simulink model "ModeSwitch_FLY"  (R2017b)
settings: Solver=FixedStepDiscrete  StartTime=0.0  StopTime=10.0  RelTol=1e-3
values from neighbouring files (symbols this model uses):
  DEG2RAD = 0.0174533    [Init_control.m]
  Kd_PITCH_AngleRate = 0.001    [Init_control.m]
  Kd_ROLL_AngleRate = 0.001    [Init_control.m]
  Kd_YAW_AngleRate = 0.00    (= 0)    [Init_control.m]
  Ki_PITCH_AngleRate = 0.02    [Init_control.m]
  Ki_ROLL_AngleRate = 0.02    [Init_control.m]
  Ki_YAW_AngleRate = 0.001    [Init_control.m]
  Kp_PITCH_ANGLE = 6.5    [Init_control.m]
  Kp_PITCH_AngleRate = 0.1    [Init_control.m]
  Kp_ROLL_ANGLE = 6.5    [Init_control.m]
  Kp_ROLL_AngleRate = 0.1    [Init_control.m]
  Kp_YAW_AngleRate = 0.3    [Init_control.m]
  Kpxp = 1.0    (= 1)    [Init_control.m]
  Kpyp = 1.0    (= 1)    [Init_control.m]
  Kpzp = 4.0    (= 4)    [Init_control.m]
  Kvxd = 0.01    [Init_control.m]
  Kvxi = 0.4    [Init_control.m]
  Kvxp = 2.5    [Init_control.m]
  Kvyd = 0.01    [Init_control.m]
  Kvyi = 0.4    [Init_control.m]
  Kvyp = 2.5    [Init_control.m]
  Kvzd = 0.005    [Init_control.m]
  Kvzi = 0.01    [Init_control.m]
  Kvzp = 0.45    [Init_control.m]
  MAX_CONTROL_ANGLE_PITCH = 35    [Init_control.m]
  MAX_CONTROL_ANGLE_RATE_PITCH = 220    [Init_control.m]
  MAX_CONTROL_ANGLE_RATE_ROLL = 220    [Init_control.m]
  MAX_CONTROL_ANGLE_RATE_Y = 200    [Init_control.m]
  MAX_CONTROL_ANGLE_ROLL = 35    [Init_control.m]
  MAX_CONTROL_VELOCITY_XY = 5    [Init_control.m]
  MAX_CONTROL_VELOCITY_Z = 3    [Init_control.m]
  Saturation_I_ah = 3.43    [Init_control.m]
  Saturation_I_az = 5    [Init_control.m]
  Saturation_I_RP_Max = 0.3    [Init_control.m]
  Saturation_I_RP_Min = -0.3    [Init_control.m]
  Saturation_I_Y_Max = 0.2    [Init_control.m]
  Saturation_I_Y_Min = -0.2    [Init_control.m]
  THR_HOVER = 0.609    [Init_control.m]
undefined symbols (not defined in the file or in its folder): DiscIntNeverNeededParam, RGBLED_COLOR_ENUM, RGBLED_MODE_ENUM
libraries: simulink x7, pixhawk_slib_sensors_actuators x5, pixhawk_slib_uORB_RW x1
settings Model: Creator=wsh  LastModifiedBy=Mr Wang
settings OptimizationCC: DefaultParameterBehavior=Inlined  MaxStackSize=64
settings DebuggingCC: ParameterTunabilityLossMsg=error
settings HardwareCC: ProdBitPerPointer=32  ProdBitPerSizeT=32  ProdBitPerPtrDiffT=32  ProdLargestAtomicInteger=Long  ProdLargestAtomicFloat=Double  ProdWordSize=32  ProdHWDeviceType=ARM Compatible->ARM Cortex
settings SFSimCC: MATLABDynamicMemAlloc=off
settings RTWCC: SystemTargetFile=ert.tlc  HardwareBoard=Pixhawk PX4  TemplateMakefile=ert_default_tmf  GenerateReport=on  Toolchain=Pixhawk Toolchain  IncludeHyperlinkInReport=on  LaunchReport=on  GenerateTraceInfo=on  GenerateTraceReport=on  GenerateTraceReportSl=on  GenerateTraceReportSf=on  GenerateTraceReportEml=on
settings CodeAppCC: ForceParamTrailComments=on  IgnoreCustomStorageClasses=off  OperatorAnnotations=on  SimulinkDataObjDesc=on  SFDataObjDesc=on  MATLABFcnDesc=on  InsertBlockDesc=on  StateflowObjectComments=on  MATLABSourceComments=on
settings ERTTargetCC: MultiwordLength=2048  ERTCustomFileTemplate=PX4_codertarget_file_process.tlc

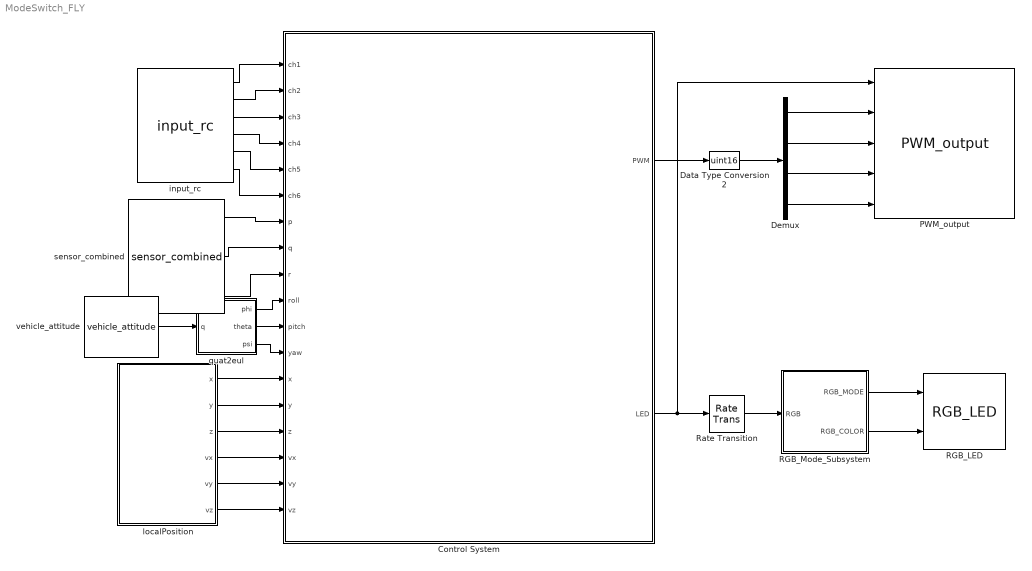
== system ModeSwitch_FLY ==
  Control System : Subsystem
      mask Display: image('icon\pixhawk.png');
  Data Type Conversion2 : DataTypeConversion  OutDataTypeStr=uint16
  Demux : Demux
  PWM_output : pixhawk_slib_sensors_actuators/PWM_output  Description=|  pub_outputs=on  pwm_rate=400Hz  show_pwm1=on  show_pwm5=off  show_pwm2=on  show_pwm6=off  show_pwm3=on  show_pwm7=off  show_pwm4=on  show_pwm8=off
      | This block allows the user to send the appropriate PWM signals out to the PX4 outputs.  
      | These are usually connected to the ESCs which control the motor speeds. 
      | In order for the flight control to arm (enable) the output from the software side, the ARM Output input must be held high (boolean TRUE).  
      | Only then will the PWM values be sent out the PX4 hardware ports.  
      | This is usually a function of the RC Tx in combination with other flight modes programmed in the Simulink model by the user.  
      | The block has 8 available ports (data type uint16) which can be selectively chosen.  
      | These correspond to the 8 PWM output ports on the px4fmu hardware.
      settings: SourceProductName=Pixhawk Target Blocks
  RGB_LED : pixhawk_slib_sensors_actuators/RGB_LED
      settings: SourceProductName=Pixhawk Target Blocks
  RGB_Mode_Subsystem : Subsystem
  Rate Transition : RateTransition  OutPortSampleTime=1
  input_rc : pixhawk_slib_sensors_actuators/input_rc  Description=|  sampletime=0.004  channel1=on  channel2=on  channel3=on  channel4=on  channel5=on  channel6=on  channel7=off  channel8=off  channel9=off  channel10=off  channel11=off  channel12=off  channel13=off  channel14=off  channel15=off  channel16=off  channel17=off  channel18=off  ch_count=off  rssi=off  rc_failsafe=off  rc_lost=off  rc_inputsource=off
      | RC Input Block
      | 
      | This block provides user input control to the model.
      | It uses the input_rc uORB topic.
      | 
      | The user has the ability to choose which channels are available as outputs from this block and also some optional outputs. These include 
      | Channels 1 through 18
      | double data type indicating the PWM value from the controller 
      | measured pulse widths for each of the supported channels 
      | Channel Count 
      | uint32 data type of the number of channels which are detector by the PX4 
      | RC Failsafe 
      | boolean data types indicating that the RC Tx is sending the FailSafe signal (if equipped and properly setup) 
      | explicit failsafe flag: true on TX failure or TX out of range , false otherwise. 
      | Only the true state is reliable, as there are some (PPM) receivers on the market going into failsafe without telling us explicitly. 
      | RC Input Source 
      | Enumeration data type indicating which source the RC input is from. 
      | Valid values are found in the ENUM file: RC_INPUT_SOURCE_ENUM.m 
      |           Enumeration members for class 'RC_INPUT_SOURCE_ENUM':
      |           RCINPUT_SOURCE_UNKNOWN         (0)
      |           RCINPUT_SOURCE_PX4FMU_PPM      (1)
      |           RCINPUT_SOURCE_PX4IO_PPM       (2)
      |           RCINPUT_SOURCE_PX4IO_SPEKTRUM  (3)
      |           RCINPUT_SOURCE_PX4IO_SBUS      (4)
      |           RCINPUT_SOURCE_PX4IO_ST24      (5)
      |           RCINPUT_SOURCE_MAVLINK         (6)
      |           RCINPUT_SOURCE_QURT            (7)
      |           RCINPUT_SOURCE_PX4FMU_SPEKTRUM (8)
      |           RCINPUT_SOURCE_PX4FMU_SBUS     (9)
      |           RCINPUT_SOURCE_PX4FMU_ST24     (10)
      |           RCINPUT_SOURCE_PX4FMU_SUMD     (11)
      |           RCINPUT_SOURCE_PX4FMU_DSM      (12)
      |           RCINPUT_SOURCE_PX4IO_SUMD      (13)
      | 
      | RSSI - Receive signal strength index 
      | receive signal strength indicator (RSSI): < 0: Undefined, 0: no signal, 255: full reception 
      | RC Lost Connection 
      | boolean data type indicating RC receiver connection status 
      | True, if no frame has arrived in the expected time, false otherwise. 
      | True usally means that the receiver has been disconnected, but can also indicate a radio link loss on "stupid" systems. 
      | Will remain false, if a RX with failsafe option continues to transmit frames after a link loss. 
      |   
      | Sample Model: px4demo_input_rc.slx
      settings: SourceProductName=Pixhawk Target Blocks
  "localPosition " : Subsystem
  quat2eul : MATLAB Function  TreatAsAtomicUnit=on
  sensor_combined : pixhawk_slib_sensors_actuators/sensor_combined  Description=|  sampletime=0.004  show_mag=off  show_acc=off  show_gyro=on  show_baro=off  show_ts=off
      | Sensor Combined Block
      | 
      | This block enables access to the various sensors available on the px4fmu-v2 hardware.  
      | The user can use these signals in the Simulink control model.  
      | The sample time needs to be provided in the mask dialog.  
      | Optional output ports can also be selected.  
      | Refer to the sample model: px4demo_attitude_control.slx
      | 
      | Signal definitions: 
      | Magnetometer (x,y,z) - single values – Magnetic field in NED body frame, in Gauss 
      | Accelerometer (x,y,z) - single values – Acceleration in NED body frame, in m/s^2 
      | Gyroscope (p,q,r) - single values – Angular velocity in radians per second 
      | Barometer (Altitude) - single value – Barometric pressure, already temperature compensated (millibars) 
      | RunTime (timestamp) - double value – Timestamp in microseconds since boot, from gyro 
      |   
      | The sensor_combined block needs to have the px4io service running on the PX4 hardware in order to get valid signal values.
      settings: SourceProductName=Pixhawk Target Blocks
  vehicle_attitude : pixhawk_slib_sensors_actuators/vehicle_attitude  Description=|  sampletime=0.004  show_r=off  show_p=off  show_y=off  show_q=on  show_ts=off
      | This block gives access to the running service that calculates the vehicle’s attitude.  A uORB topic (vehicle_attitude (attitude measurements)) publisher MUST be running in order for this block to provide valid signal values.  The available ones as of v1.3 are: 
      | attitude_estimator_ekf – EKF-Extended Kalman Filter for attitude estimation 
      | attitude_estimator_so3 – SO(3)-attitude estimation by using accelerometer, gyroscopes and magnetometer 
      | One of these MUST be running on the px4fmu in order for this block to return valid values.  Refer to the sample model: px4demo_attitude_control.slx. Attitude in NED (North-East-Down) body frame in SI units. 
      | Signal definitions: 
      | Roll – single value, Roll angle (rad, Tait-Bryan, NED) 
      | Pitch – single value, Pitch angle (rad, Tait-Bryan, NED) 
      | Yaw – single value, Yaw angle (rad, Tait-Bryan, NED) 
      | Quaternion (NED) – single(4) values (optional based on the uORB publisher)
      settings: SourceProductName=Pixhawk Target Blocks
  wires:
  sensor_combined/1 -> Control System/7(p)
  sensor_combined/3 -> Control System/9(r)
  quat2eul/1(phi) -> Control System/10(roll)
  quat2eul/2(theta) -> Control System/11(pitch)
  sensor_combined/2 -> Control System/8(q)
  Control System/1(PWM) -> Data Type Conversion2/1
  quat2eul/3(psi) -> Control System/12(yaw)
  "localPosition "/1(x) -> Control System/13(x)
  "localPosition "/2(y) -> Control System/14(y)
  "localPosition "/3(z) -> Control System/15(z)
  "localPosition "/4(vx) -> Control System/16(vx)
  "localPosition "/5(vy) -> Control System/17(vy)
  "localPosition "/6(vz) -> Control System/18(vz)
  input_rc/4 -> Control System/4(ch4)
  input_rc/3 -> Control System/3(ch3)
  input_rc/2 -> Control System/2(ch2)
  input_rc/1 -> Control System/1(ch1)
  input_rc/5 -> Control System/5(ch5)
  input_rc/6 -> Control System/6(ch6)
  vehicle_attitude/1 -> quat2eul/1(q)
  RGB_Mode_Subsystem/2(RGB_COLOR) -> RGB_LED/2
  Rate Transition/1 -> RGB_Mode_Subsystem/1(RGB)
  Control System/2(LED) -> PWM_output/1, Rate Transition/1
  RGB_Mode_Subsystem/1(RGB_MODE) -> RGB_LED/1
  Data Type Conversion2/1 -> Demux/1
  Demux/1 -> PWM_output/2
  Demux/2 -> PWM_output/3
  Demux/3 -> PWM_output/4
  Demux/4 -> PWM_output/5

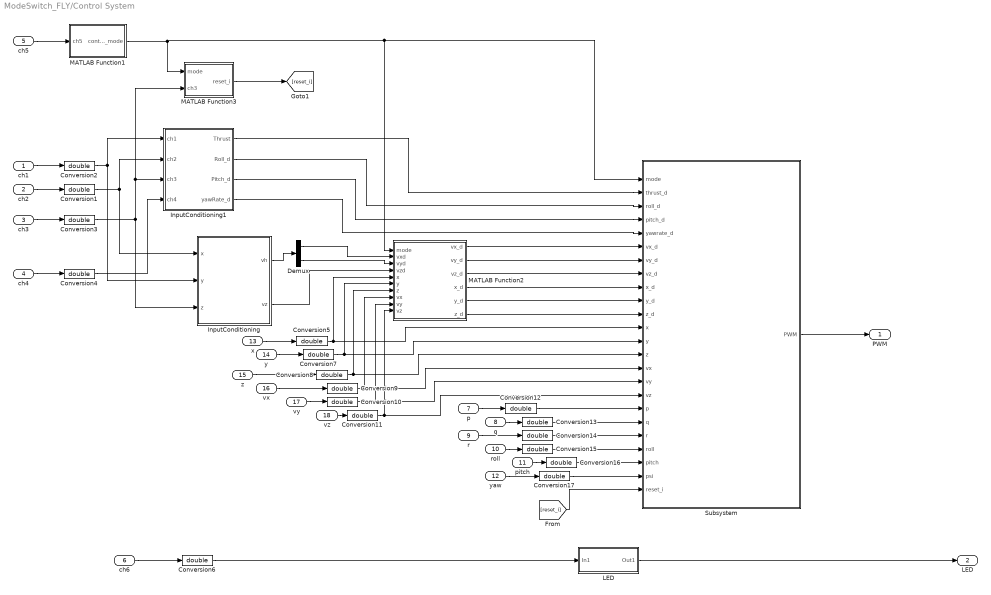
== system ModeSwitch_FLY/Control System ==
  ch1 : Inport  OutDataTypeStr=uint16  PortDimensions=1
  ch2 : Inport  Port=2  OutDataTypeStr=uint16  PortDimensions=1
  ch3 : Inport  Port=3  OutDataTypeStr=uint16  PortDimensions=1
  ch4 : Inport  Port=4  OutDataTypeStr=uint16  PortDimensions=1
  ch5 : Inport  Port=5  OutDataTypeStr=uint16  PortDimensions=1  Interpolate=off
  ch6 : Inport  Port=6  OutDataTypeStr=uint16  PortDimensions=1  Interpolate=off
  p : Inport  Port=7  PortDimensions=1
  q : Inport  Port=8  PortDimensions=1
  r : Inport  Port=9  PortDimensions=1
  roll : Inport  Port=10  PortDimensions=1
  pitch : Inport  Port=11  PortDimensions=1
  yaw : Inport  Port=12  PortDimensions=1
  x : Inport  Port=13
  y : Inport  Port=14
  z : Inport  Port=15
  vx : Inport  Port=16
  vy : Inport  Port=17
  vz : Inport  Port=18
  Conversion{1..17} (17 alike) : DataTypeConversion  OutDataTypeStr=double
  Demux : Demux  Outputs=2
  InputConditioning : Subsystem
  InputConditioning1 : Subsystem
  "LED " : Subsystem
  MATLAB Function1 : MATLAB Function  TreatAsAtomicUnit=on
  MATLAB Function2 : MATLAB Function  TreatAsAtomicUnit=on
  MATLAB Function3 : MATLAB Function  TreatAsAtomicUnit=on
  Subsystem : Subsystem
  PWM : Outport
  LED : Outport  Port=2  PortDimensions=1
  wires:
  ch3/1 -> Conversion3/1
  ch6/1 -> Conversion6/1
  ch4/1 -> Conversion4/1
  "LED "/1(Out1) -> LED/1
  Conversion6/1 -> "LED "/1(In1)
  Conversion4/1 -> InputConditioning1/4(ch4)
  ch1/1 -> Conversion2/1
  ch2/1 -> Conversion1/1
  Conversion1/1 -> InputConditioning1/2(ch2), InputConditioning/1(x)
  x/1 -> Conversion5/1
  y/1 -> Conversion7/1
  z/1 -> Conversion8/1
  MATLAB Function1/1(control_mode) -> MATLAB Function3/1(mode), Subsystem/1(mode), MATLAB Function2/1(mode)
  roll/1 -> Conversion15/1
  pitch/1 -> Conversion16/1
  p/1 -> Conversion12/1
  q/1 -> Conversion13/1
  r/1 -> Conversion14/1
  yaw/1 -> Conversion17/1
  vz/1 -> Conversion11/1
  vy/1 -> Conversion10/1
  vx/1 -> Conversion9/1
  InputConditioning1/2(Roll_d) -> Subsystem/3(roll_d)
  InputConditioning1/3(Pitch_d) -> Subsystem/4(pitch_d)
  InputConditioning1/1(Thrust) -> Subsystem/2(thrust_d)
  InputConditioning1/4(yawRate_d) -> Subsystem/5(yawrate_d)
  Conversion5/1 -> Subsystem/12(x), MATLAB Function2/5(x)
  Conversion7/1 -> Subsystem/13(y), MATLAB Function2/6(y)
  Conversion8/1 -> Subsystem/14(z), MATLAB Function2/7(z)
  Conversion9/1 -> Subsystem/15(vx), MATLAB Function2/8(vx)
  Conversion10/1 -> Subsystem/16(vy), MATLAB Function2/9(vy)
  Conversion11/1 -> Subsystem/17(vz), MATLAB Function2/10(vz)
  Conversion12/1 -> Subsystem/18(p)
  Conversion13/1 -> Subsystem/19(q)
  Conversion14/1 -> Subsystem/20(r)
  Conversion15/1 -> Subsystem/21(roll)
  Conversion16/1 -> Subsystem/22(pitch)
  Conversion17/1 -> Subsystem/23(psi)
  [reset_i] -> Subsystem/24(reset_i)
  Conversion2/1 -> InputConditioning1/1("ch1 "), InputConditioning/2(y)
  InputConditioning/2(vz) -> MATLAB Function2/4(vzd)
  MATLAB Function2/1(vx_d) -> Subsystem/6(vx_d)
  MATLAB Function2/2(vy_d) -> Subsystem/7(vy_d)
  MATLAB Function2/3(vz_d) -> Subsystem/8(vz_d)
  MATLAB Function2/4(x_d) -> Subsystem/9(x_d)
  MATLAB Function2/5(y_d) -> Subsystem/10(y_d)
  MATLAB Function2/6(z_d) -> Subsystem/11(z_d)
  InputConditioning/1(vh) -> Demux/1
  Demux/1 -> MATLAB Function2/2(vxd)
  Demux/2 -> MATLAB Function2/3(vyd)
  Conversion3/1 -> InputConditioning/3(z), InputConditioning1/3(ch3), MATLAB Function3/2(ch3)
  ch5/1 -> MATLAB Function1/1(ch5)
  MATLAB Function3/1(reset_i) -> [reset_i]
  Subsystem/1(PWM) -> PWM/1

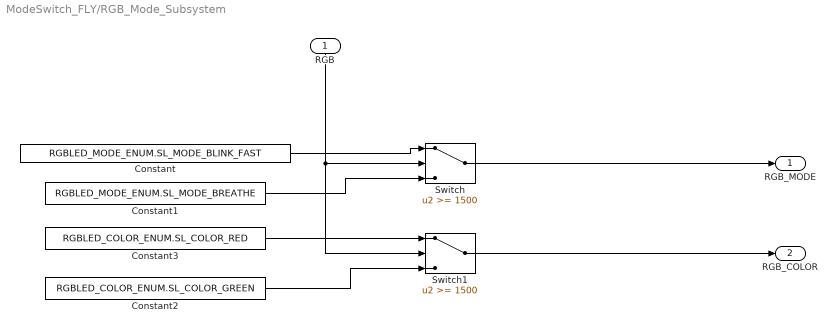
== system ModeSwitch_FLY/RGB_Mode_Subsystem ==
  RGB : Inport
  Constant : Constant  Value=RGBLED_MODE_ENUM.SL_MODE_BLINK_FAST  OutDataTypeStr=Enum: RGBLED_MODE_ENUM
  Constant1 : Constant  Value=RGBLED_MODE_ENUM.SL_MODE_BREATHE  OutDataTypeStr=Enum: RGBLED_MODE_ENUM
  Constant2 : Constant  Value=RGBLED_COLOR_ENUM.SL_COLOR_GREEN  OutDataTypeStr=Enum: RGBLED_COLOR_ENUM
  Constant3 : Constant  Value=RGBLED_COLOR_ENUM.SL_COLOR_RED  OutDataTypeStr=Enum: RGBLED_COLOR_ENUM
  Switch : Switch  Threshold=1500
  Switch1 : Switch  Threshold=1500
  RGB_MODE : Outport
  RGB_COLOR : Outport  Port=2
  wires:
  RGB/1 -> Switch1/2, Switch/2
  Constant/1 -> Switch/1
  Constant1/1 -> Switch/3
  Switch/1 -> RGB_MODE/1
  Constant3/1 -> Switch1/1
  Constant2/1 -> Switch1/3
  Switch1/1 -> RGB_COLOR/1

== system ModeSwitch_FLY/localPosition  ==
  Bus Selector2 : BusSelector  OutputSignals=x,y,z,vx,vy,vz
  uORB Read Function-Call Trigger : pixhawk_slib_uORB_RW/uORB Read Function-Call Trigger  uORB_Topic_str='vehicle_local_position'  BusObjVar=Bus: vehicle_local_position_SL  uORB_Interval=1  AsyncOutput=off  Fcn_call_select=Generate Function Call Signal  TaskName='Task1'  Poll_timeout=100  Ts=-1
      settings: SourceProductName=Pixhawk Target Blocks
  x : Outport
  y : Outport  Port=2
  z : Outport  Port=3
  vx : Outport  Port=4
  vy : Outport  Port=5
  vz : Outport  Port=6
  wires:
  Bus Selector2/3 -> z/1  "<z>"
  Bus Selector2/2 -> y/1  "<y>"
  Bus Selector2/1 -> x/1  "<x>"
  Bus Selector2/4 -> vx/1  "<vx>"
  Bus Selector2/5 -> vy/1  "<vy>"
  Bus Selector2/6 -> vz/1  "<vz>"
  uORB Read Function-Call Trigger/1 -> Bus Selector2/1

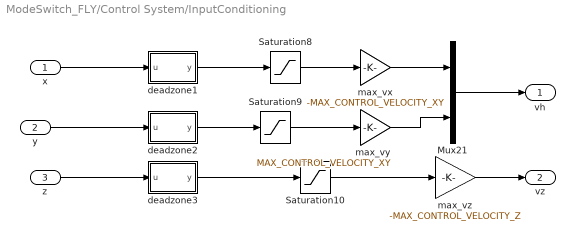
== system ModeSwitch_FLY/Control System/InputConditioning ==
  x : Inport
  y : Inport  Port=2
  z : Inport  Port=3
  Mux21 : Mux  Inputs=2
  Saturation10 : Saturate  UpperLimit=1  LowerLimit=-1
  Saturation8 : Saturate  UpperLimit=1  LowerLimit=-1
  Saturation9 : Saturate  UpperLimit=1  LowerLimit=-1
  deadzone1 : MATLAB Function  TreatAsAtomicUnit=on
  deadzone2 : MATLAB Function  TreatAsAtomicUnit=on
  deadzone3 : MATLAB Function  TreatAsAtomicUnit=on
  max_vx : Gain  Gain=-MAX_CONTROL_VELOCITY_XY  OutDataTypeStr=Inherit: Inherit via back propagation
  max_vy : Gain  Gain=MAX_CONTROL_VELOCITY_XY  OutDataTypeStr=Inherit: Inherit via back propagation
  max_vz : Gain  Gain=-MAX_CONTROL_VELOCITY_Z  OutDataTypeStr=Inherit: Inherit via back propagation
  vh : Outport
  vz : Outport  Port=2
  wires:
  Saturation10/1 -> max_vz/1
  Mux21/1 -> vh/1
  Saturation8/1 -> max_vx/1
  deadzone3/1(y) -> Saturation10/1
  deadzone2/1(y) -> Saturation9/1
  deadzone1/1(y) -> Saturation8/1
  Saturation9/1 -> max_vy/1
  x/1 -> deadzone1/1(u)
  z/1 -> deadzone3/1(u)
  y/1 -> deadzone2/1(u)
  max_vz/1 -> vz/1
  max_vx/1 -> Mux21/1
  max_vy/1 -> Mux21/2

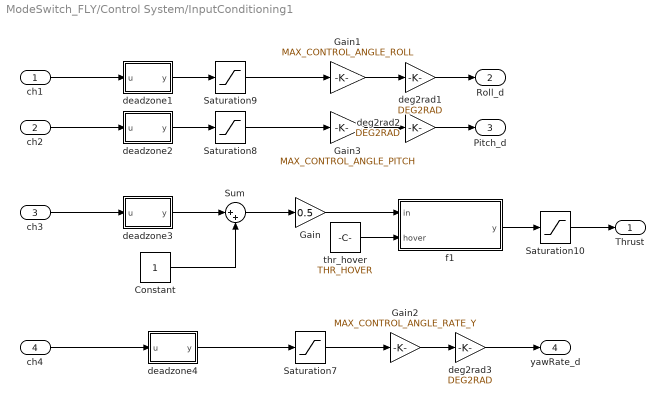
== system ModeSwitch_FLY/Control System/InputConditioning1 ==
  "ch1 " : Inport
  ch2 : Inport  Port=2
  ch3 : Inport  Port=3
  ch4 : Inport  Port=4
  Constant : Constant
  Gain : Gain  Gain=0.5
  Gain1 : Gain  Gain=MAX_CONTROL_ANGLE_ROLL  OutDataTypeStr=Inherit: Inherit via back propagation
  Gain2 : Gain  Gain=MAX_CONTROL_ANGLE_RATE_Y
  Gain3 : Gain  Gain=MAX_CONTROL_ANGLE_PITCH  OutDataTypeStr=Inherit: Inherit via back propagation
  Saturation10 : Saturate  UpperLimit=1  LowerLimit=0
  Saturation7 : Saturate  UpperLimit=1  LowerLimit=-1
  Saturation8 : Saturate  UpperLimit=1  LowerLimit=-1
  Saturation9 : Saturate  UpperLimit=1  LowerLimit=-1
  Sum : Sum  Inputs=|++
  deadzone1 : MATLAB Function  TreatAsAtomicUnit=on
  deadzone2 : MATLAB Function  TreatAsAtomicUnit=on
  deadzone3 : MATLAB Function  TreatAsAtomicUnit=on
  deadzone4 : MATLAB Function  TreatAsAtomicUnit=on
  deg2rad1 : Gain  Gain=DEG2RAD
  deg2rad2 : Gain  Gain=DEG2RAD
  deg2rad3 : Gain  Gain=DEG2RAD
  f1 : MATLAB Function  TreatAsAtomicUnit=on
  "thr_hover " : Constant  Value=THR_HOVER
  Thrust : Outport
  Roll_d : Outport  Port=2
  Pitch_d : Outport  Port=3
  yawRate_d : Outport  Port=4
  wires:
  deadzone3/1(y) -> Sum/1
  ch3/1 -> deadzone3/1(u)
  deadzone2/1(y) -> Saturation8/1
  Saturation10/1 -> Thrust/1
  deadzone1/1(y) -> Saturation9/1
  "ch1 "/1 -> deadzone1/1(u)
  ch2/1 -> deadzone2/1(u)
  Saturation9/1 -> Gain1/1
  Saturation8/1 -> Gain3/1
  Gain3/1 -> deg2rad2/1
  Constant/1 -> Sum/2
  Sum/1 -> Gain/1
  Gain1/1 -> deg2rad1/1
  deg2rad1/1 -> Roll_d/1
  deg2rad2/1 -> Pitch_d/1
  Saturation7/1 -> Gain2/1
  deadzone4/1(y) -> Saturation7/1
  ch4/1 -> deadzone4/1(u)
  Gain2/1 -> deg2rad3/1
  deg2rad3/1 -> yawRate_d/1
  "thr_hover "/1 -> f1/2(hover)
  Gain/1 -> f1/1(in)
  f1/1(y) -> Saturation10/1

== system ModeSwitch_FLY/Control System/LED  ==
  In1 : Inport
  Compare To Constant3 : simulink/Logic and Bit Operations/Compare To Constant  relop=>=  const=uint16(1500)  OutDataTypeStr=boolean
  Out1 : Outport
  wires:
  Compare To Constant3/1 -> Out1/1
  In1/1 -> Compare To Constant3/1

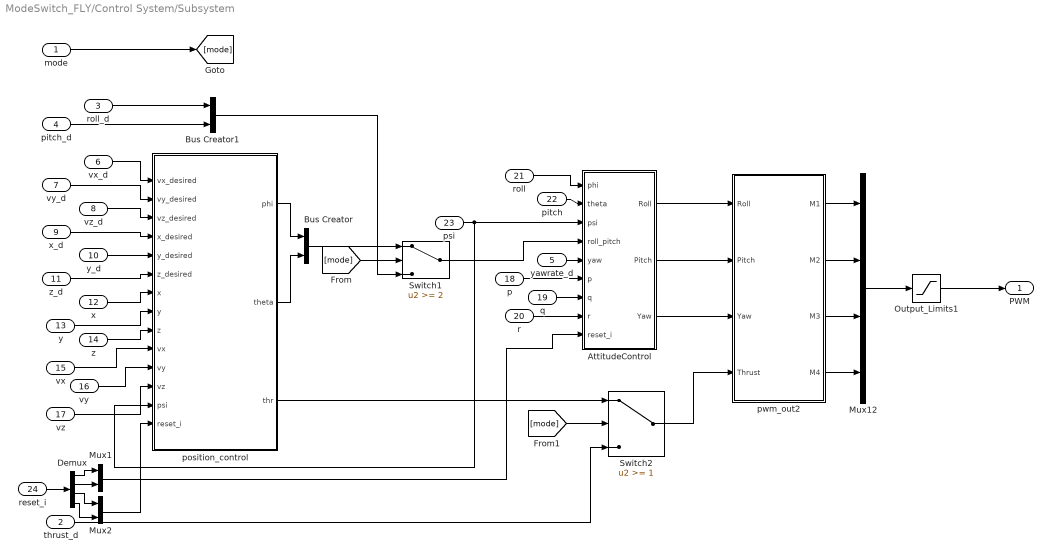
== system ModeSwitch_FLY/Control System/Subsystem ==
  mode : Inport
  thrust_d : Inport  Port=2
  roll_d : Inport  Port=3
  pitch_d : Inport  Port=4
  yawrate_d : Inport  Port=5
  vx_d : Inport  Port=6
  vy_d : Inport  Port=7
  vz_d : Inport  Port=8
  x_d : Inport  Port=9
  y_d : Inport  Port=10
  z_d : Inport  Port=11
  x : Inport  Port=12
  y : Inport  Port=13
  z : Inport  Port=14
  vx : Inport  Port=15
  vy : Inport  Port=16
  vz : Inport  Port=17
  p : Inport  Port=18  PortDimensions=1
  q : Inport  Port=19  PortDimensions=1
  r : Inport  Port=20  PortDimensions=1
  roll : Inport  Port=21  PortDimensions=1
  pitch : Inport  Port=22  PortDimensions=1
  psi : Inport  Port=23  PortDimensions=1
  reset_i : Inport  Port=24
  AttitudeControl : Subsystem
  Bus Creator : BusCreator  Inputs=2
  Bus Creator1 : BusCreator  Inputs=2
  Demux : Demux
  Mux1 : Mux  Inputs=2
  Mux12 : Mux
  Mux2 : Mux  Inputs=2
  Output_Limits1 : Saturate  UpperLimit=2000  LowerLimit=1000
  Switch1 : Switch  Threshold=2
  Switch2 : Switch  Threshold=1
  position_control : Subsystem
  pwm_out2 : MATLAB Function  SystemSampleTime=0.004
  PWM : Outport
  wires:
  pwm_out2/4(M4) -> Mux12/4
  pwm_out2/3(M3) -> Mux12/3
  yawrate_d/1 -> AttitudeControl/5(yaw)
  roll/1 -> AttitudeControl/1(phi)
  Output_Limits1/1 -> PWM/1
  q/1 -> AttitudeControl/7(q)
  AttitudeControl/1(Roll) -> pwm_out2/1(Roll)
  pwm_out2/2(M2) -> Mux12/2
  AttitudeControl/2(Pitch) -> pwm_out2/2(Pitch)
  pitch/1 -> AttitudeControl/2(theta)
  Mux12/1 -> Output_Limits1/1
  position_control/2(theta) -> Bus Creator/2
  pwm_out2/1(M1) -> Mux12/1
  AttitudeControl/3(Yaw) -> pwm_out2/3(Yaw)
  position_control/1(phi) -> Bus Creator/1
  p/1 -> AttitudeControl/6(p)
  vx/1 -> position_control/10(vx)
  vz/1 -> position_control/12(vz)
  vy/1 -> position_control/11(vy)
  x_d/1 -> position_control/4(x_desired)
  y_d/1 -> position_control/5(y_desired)
  z_d/1 -> position_control/6(z_desired)
  mode/1 -> [mode]
  vz_d/1 -> position_control/3(vz_desired)
  x/1 -> position_control/7(x)
  vx_d/1 -> position_control/1(vx_desired)
  vy_d/1 -> position_control/2(vy_desired)
  y/1 -> position_control/8(y)
  z/1 -> position_control/9(z)
  Bus Creator/1 -> Switch1/1
  [mode] -> Switch1/2
  Switch1/1 -> AttitudeControl/4(roll_pitch)
  roll_d/1 -> Bus Creator1/1
  pitch_d/1 -> Bus Creator1/2
  Bus Creator1/1 -> Switch1/3
  [mode] -> Switch2/2
  position_control/3(thr) -> Switch2/1
  Switch2/1 -> pwm_out2/4(Thrust)
  thrust_d/1 -> Switch2/3
  r/1 -> AttitudeControl/8(r)
  psi/1 -> AttitudeControl/3(psi), position_control/13(psi)
  reset_i/1 -> Demux/1
  Mux2/1 -> position_control/14(reset_i)
  Mux1/1 -> AttitudeControl/9(reset_i)
  Demux/1 -> Mux1/1
  Demux/2 -> Mux1/2
  Demux/3 -> Mux2/1
  Demux/4 -> Mux2/2

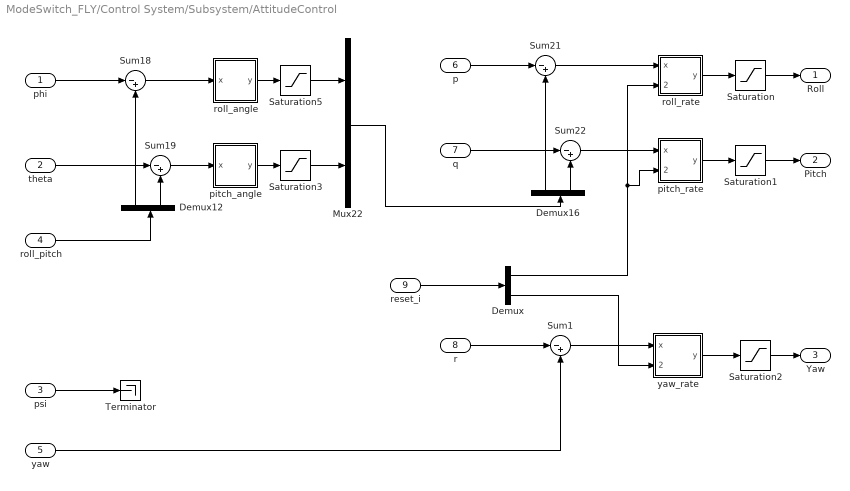
== system ModeSwitch_FLY/Control System/Subsystem/AttitudeControl ==
  phi : Inport
  theta : Inport  Port=2
  psi : Inport  Port=3
  roll_pitch : Inport  Port=4
  yaw : Inport  Port=5
  p : Inport  Port=6
  q : Inport  Port=7
  r : Inport  Port=8
  reset_i : Inport  Port=9
  Demux : Demux  Outputs=2
  Demux12 : Demux  Outputs=2
  Demux16 : Demux  Outputs=2
  Mux22 : Mux  Inputs=2
  Saturation : Saturate  UpperLimit=1  LowerLimit=-1
  Saturation1 : Saturate  UpperLimit=1  LowerLimit=-1
  Saturation2 : Saturate
  Saturation3 : Saturate  UpperLimit=MAX_CONTROL_ANGLE_RATE_PITCH  LowerLimit=-MAX_CONTROL_ANGLE_RATE_PITCH
  Saturation5 : Saturate  UpperLimit=MAX_CONTROL_ANGLE_RATE_ROLL  LowerLimit=-MAX_CONTROL_ANGLE_RATE_ROLL
  Sum1 : Sum  Inputs=|-+
  Sum18 : Sum  Inputs=|-+  OutMin=-90  OutMax=90
  Sum19 : Sum  Inputs=|-+  OutMin=-90  OutMax=90
  Sum21 : Sum  Inputs=|-+
  Sum22 : Sum  Inputs=|-+
  Terminator : Terminator
  "pitch_angle " : Subsystem
  pitch_rate : Subsystem
  "roll_angle " : Subsystem
  roll_rate : Subsystem
  yaw_rate : Subsystem
  Roll : Outport
  Pitch : Outport  Port=2
  Yaw : Outport  Port=3
  wires:
  Sum19/1 -> "pitch_angle "/1(x)
  "pitch_angle "/1(y) -> Saturation3/1
  Demux12/1 -> Sum18/2
  Demux12/2 -> Sum19/2
  phi/1 -> Sum18/1
  theta/1 -> Sum19/1
  Sum18/1 -> "roll_angle "/1(x)
  Sum22/1 -> pitch_rate/1(x)
  p/1 -> Sum21/1
  q/1 -> Sum22/1
  Sum21/1 -> roll_rate/1(x)
  Demux16/1 -> Sum21/2
  pitch_rate/1(y) -> Saturation1/1
  roll_rate/1(y) -> Saturation/1
  yaw_rate/1(y) -> Saturation2/1
  roll_pitch/1 -> Demux12/1
  Saturation/1 -> Roll/1
  Saturation1/1 -> Pitch/1
  Saturation2/1 -> Yaw/1
  Demux16/2 -> Sum22/2
  Mux22/1 -> Demux16/1
  r/1 -> Sum1/1
  Sum1/1 -> yaw_rate/1(x)
  "roll_angle "/1(y) -> Saturation5/1
  Saturation5/1 -> Mux22/1
  Saturation3/1 -> Mux22/2
  yaw/1 -> Sum1/2
  Demux/1 -> roll_rate/2(reset_i), pitch_rate/2(reset_i)
  reset_i/1 -> Demux/1
  Demux/2 -> yaw_rate/2(reset_i)
  psi/1 -> Terminator/1

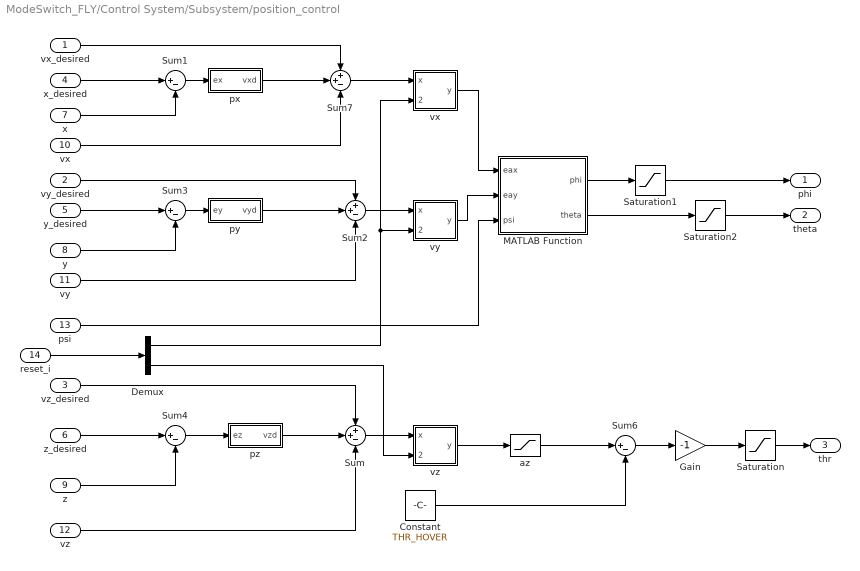
== system ModeSwitch_FLY/Control System/Subsystem/position_control ==
  vx_desired : Inport
  vy_desired : Inport  Port=2
  vz_desired : Inport  Port=3
  x_desired : Inport  Port=4
  y_desired : Inport  Port=5
  z_desired : Inport  Port=6
  x : Inport  Port=7
  y : Inport  Port=8
  z : Inport  Port=9
  vx : Inport  Port=10
  vy : Inport  Port=11
  vz : Inport  Port=12
  psi : Inport  Port=13
  reset_i : Inport  Port=14
  Constant : Constant  Value=THR_HOVER
  Demux : Demux  Outputs=2
  Gain : Gain  Gain=-1
  MATLAB Function : MATLAB Function  TreatAsAtomicUnit=on
  Saturation : Saturate  UpperLimit=0.9  LowerLimit=0
  Saturation1 : Saturate  UpperLimit=MAX_CONTROL_ANGLE_ROLL*DEG2RAD  LowerLimit=-MAX_CONTROL_ANGLE_ROLL*DEG2RAD
  Saturation2 : Saturate  UpperLimit=MAX_CONTROL_ANGLE_PITCH*DEG2RAD/2  LowerLimit=-MAX_CONTROL_ANGLE_PITCH*DEG2RAD/2
  Sum : Sum  Inputs=++-
  Sum{1,3..4,6} (4 alike) : Sum  Inputs=|+-
  Sum2 : Sum  Inputs=++-
  Sum7 : Sum  Inputs=++-
  az : Saturate  UpperLimit=0.4  LowerLimit=-0.4
  px : Subsystem
  py : Subsystem
  pz : Subsystem
  "vx " : Subsystem
  "vy " : Subsystem
  "vz " : Subsystem
  phi : Outport
  theta : Outport  Port=2
  thr : Outport  Port=3
  wires:
  Saturation/1 -> thr/1
  Gain/1 -> Saturation/1
  Sum6/1 -> Gain/1
  "vz "/1(y) -> az/1
  Sum4/1 -> pz/1(ez)
  z/1 -> Sum4/2
  Constant/1 -> Sum6/2
  Sum/1 -> "vz "/1(x)
  vz/1 -> Sum/3
  vx/1 -> Sum7/3
  x/1 -> Sum1/2
  y/1 -> Sum3/2
  Sum3/1 -> py/1(ey)
  y_desired/1 -> Sum3/1
  vy/1 -> Sum2/3
  Sum2/1 -> "vy "/1(x)
  Sum7/1 -> "vx "/1(x)
  Sum1/1 -> px/1(ex)
  vy_desired/1 -> Sum2/1
  py/1(vyd) -> Sum2/2
  pz/1(vzd) -> Sum/2
  z_desired/1 -> Sum4/1
  vz_desired/1 -> Sum/1
  "vx "/1(y) -> MATLAB Function/1(eax)
  px/1(vxd) -> Sum7/2
  Saturation1/1 -> phi/1
  Saturation2/1 -> theta/1
  x_desired/1 -> Sum1/1
  vx_desired/1 -> Sum7/1
  "vy "/1(y) -> MATLAB Function/2(eay)
  psi/1 -> MATLAB Function/3(psi)
  MATLAB Function/1(phi) -> Saturation1/1
  MATLAB Function/2(theta) -> Saturation2/1
  reset_i/1 -> Demux/1
  Demux/1 -> "vy "/2(reset_i), "vx "/2(reset_i)
  Demux/2 -> "vz "/2(reset_i)
  az/1 -> Sum6/1

== system ModeSwitch_FLY/Control System/Subsystem/AttitudeControl/pitch_angle  ==
  x : Inport
  Gain : Gain  Gain=Kp_PITCH_ANGLE
  y : Outport  InitialOutput=0
  wires:
  x/1 -> Gain/1
  Gain/1 -> y/1

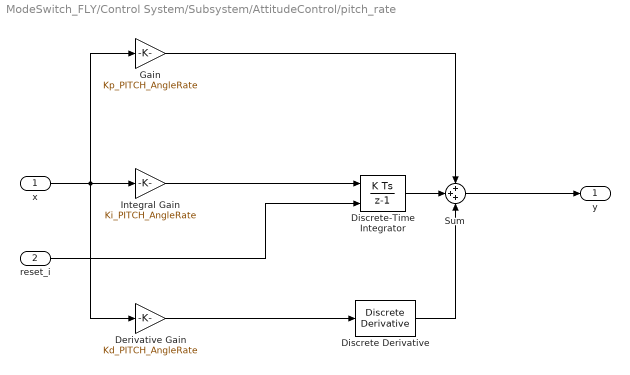
== system ModeSwitch_FLY/Control System/Subsystem/AttitudeControl/pitch_rate ==
  x : Inport
  reset_i : Inport  Port=2
  Derivative Gain : Gain  DisableCoverage=on  Gain=Kd_PITCH_AngleRate  ParamMin=-100  ParamMax=100  OutMin=-100  OutMax=100
  Discrete Derivative : simulink/Discrete/Discrete Derivative  gainval=1.0  ICPrevScaledInput=0.0  OutMin=[]  OutMax=[]  OutDataType=fixdt(1, 16)  OutScaling=2^-10  DoSatur=off
  Discrete-Time Integrator : DiscreteIntegrator  ExternalReset=level  InitialConditionSetting=State (most efficient)  SampleTime=-1  LimitOutput=on  UpperSaturationLimit=Saturation_I_RP_Max  LowerSaturationLimit=Saturation_I_RP_Min  ICPrevOutput=DiscIntNeverNeededParam  ICPrevScaledInput=DiscIntNeverNeededParam
  Gain : Gain  Gain=Kp_PITCH_AngleRate
  Integral Gain : Gain  DisableCoverage=on  Gain=Ki_PITCH_AngleRate
  Sum : Sum  Inputs=+++
  y : Outport  InitialOutput=0
  wires:
  Discrete-Time Integrator/1 -> Sum/2
  Discrete Derivative/1 -> Sum/3
  Sum/1 -> y/1
  Gain/1 -> Sum/1
  Derivative Gain/1 -> Discrete Derivative/1
  Integral Gain/1 -> Discrete-Time Integrator/1
  x/1 -> Derivative Gain/1, Integral Gain/1, Gain/1
  reset_i/1 -> Discrete-Time Integrator/2

== system ModeSwitch_FLY/Control System/Subsystem/AttitudeControl/roll_angle  ==
  x : Inport
  Gain : Gain  Gain=Kp_ROLL_ANGLE
  y : Outport  InitialOutput=0
  wires:
  Gain/1 -> y/1
  x/1 -> Gain/1

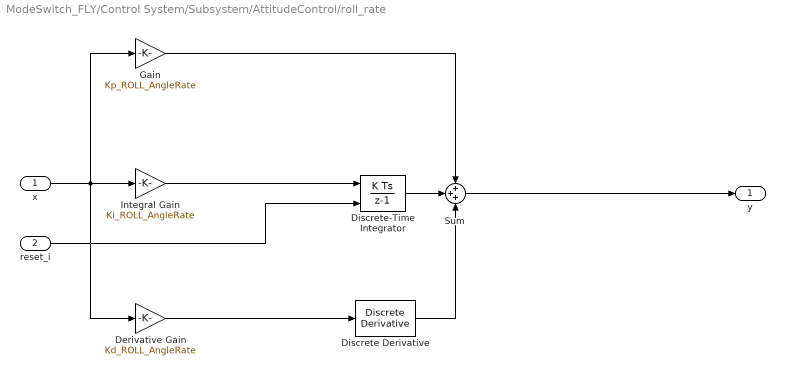
== system ModeSwitch_FLY/Control System/Subsystem/AttitudeControl/roll_rate ==
  x : Inport
  reset_i : Inport  Port=2
  Derivative Gain : Gain  DisableCoverage=on  Gain=Kd_ROLL_AngleRate  ParamMin=-100  ParamMax=100  OutMin=-100  OutMax=100
  Discrete Derivative : simulink/Discrete/Discrete Derivative  gainval=1.0  ICPrevScaledInput=0.0  OutMin=[]  OutMax=[]  OutDataType=fixdt(1, 16)  OutScaling=2^-10  DoSatur=off
  Discrete-Time Integrator : DiscreteIntegrator  ExternalReset=level  InitialConditionSetting=State (most efficient)  SampleTime=-1  LimitOutput=on  UpperSaturationLimit=Saturation_I_RP_Max  LowerSaturationLimit=Saturation_I_RP_Min  ICPrevOutput=DiscIntNeverNeededParam  ICPrevScaledInput=DiscIntNeverNeededParam
  Gain : Gain  Gain=Kp_ROLL_AngleRate
  Integral Gain : Gain  DisableCoverage=on  Gain=Ki_ROLL_AngleRate
  Sum : Sum  Inputs=+++
  y : Outport  InitialOutput=0
  wires:
  x/1 -> Gain/1, Integral Gain/1, Derivative Gain/1
  Integral Gain/1 -> Discrete-Time Integrator/1
  Derivative Gain/1 -> Discrete Derivative/1
  Gain/1 -> Sum/1
  Sum/1 -> y/1
  Discrete Derivative/1 -> Sum/3
  Discrete-Time Integrator/1 -> Sum/2
  reset_i/1 -> Discrete-Time Integrator/2

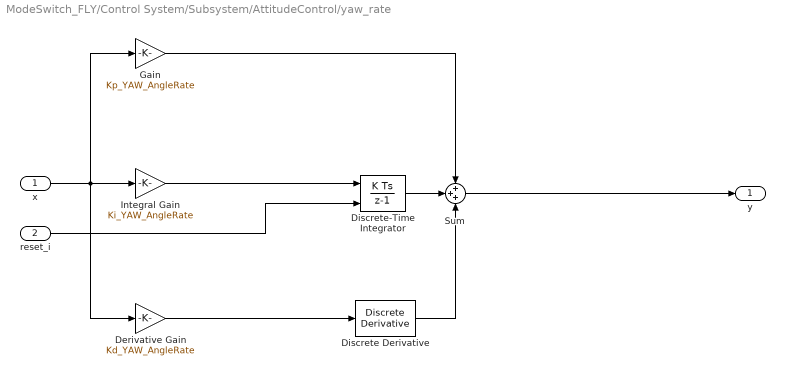
== system ModeSwitch_FLY/Control System/Subsystem/AttitudeControl/yaw_rate ==
  x : Inport
  reset_i : Inport  Port=2
  Derivative Gain : Gain  DisableCoverage=on  Gain=Kd_YAW_AngleRate  ParamMin=-100  ParamMax=100  OutMin=-100  OutMax=100
  Discrete Derivative : simulink/Discrete/Discrete Derivative  gainval=1.0  ICPrevScaledInput=0.0  OutMin=[]  OutMax=[]  OutDataType=fixdt(1, 16)  OutScaling=2^-10  DoSatur=off
  Discrete-Time Integrator : DiscreteIntegrator  ExternalReset=level  InitialConditionSetting=State (most efficient)  SampleTime=-1  LimitOutput=on  UpperSaturationLimit=Saturation_I_Y_Max  LowerSaturationLimit=Saturation_I_Y_Min  ICPrevOutput=DiscIntNeverNeededParam  ICPrevScaledInput=DiscIntNeverNeededParam
  Gain : Gain  Gain=Kp_YAW_AngleRate
  Integral Gain : Gain  DisableCoverage=on  Gain=Ki_YAW_AngleRate
  Sum : Sum  Inputs=+++
  y : Outport  InitialOutput=0
  wires:
  x/1 -> Gain/1, Integral Gain/1, Derivative Gain/1
  Integral Gain/1 -> Discrete-Time Integrator/1
  Derivative Gain/1 -> Discrete Derivative/1
  Gain/1 -> Sum/1
  Sum/1 -> y/1
  Discrete Derivative/1 -> Sum/3
  Discrete-Time Integrator/1 -> Sum/2
  reset_i/1 -> Discrete-Time Integrator/2

== system ModeSwitch_FLY/Control System/Subsystem/position_control/px ==
  ex : Inport
  Gain1 : Gain  Gain=Kpxp
  Saturation3 : Saturate  UpperLimit=MAX_CONTROL_VELOCITY_XY  LowerLimit=-MAX_CONTROL_VELOCITY_XY
  vxd : Outport
  wires:
  ex/1 -> Gain1/1
  Saturation3/1 -> vxd/1
  Gain1/1 -> Saturation3/1

== system ModeSwitch_FLY/Control System/Subsystem/position_control/py ==
  ey : Inport
  Gain1 : Gain  Gain=Kpyp
  Saturation3 : Saturate  UpperLimit=MAX_CONTROL_VELOCITY_XY  LowerLimit=-MAX_CONTROL_VELOCITY_XY
  vyd : Outport
  wires:
  Gain1/1 -> Saturation3/1
  Saturation3/1 -> vyd/1
  ey/1 -> Gain1/1

== system ModeSwitch_FLY/Control System/Subsystem/position_control/pz ==
  ez : Inport
  Gain1 : Gain  Gain=Kpzp
  Saturation3 : Saturate  UpperLimit=MAX_CONTROL_VELOCITY_Z  LowerLimit=-MAX_CONTROL_VELOCITY_Z
  vzd : Outport
  wires:
  ez/1 -> Gain1/1
  Saturation3/1 -> vzd/1
  Gain1/1 -> Saturation3/1

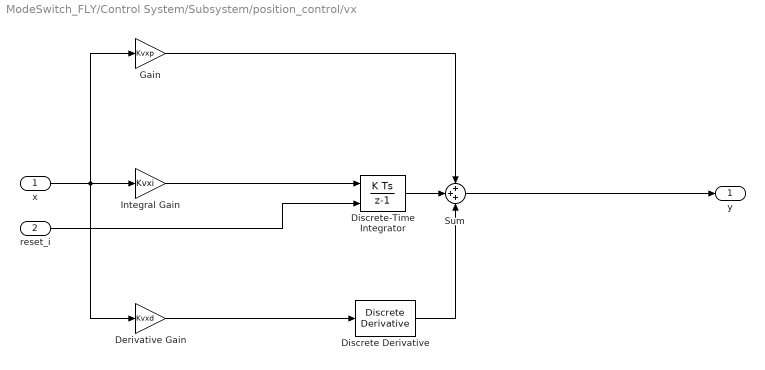
== system ModeSwitch_FLY/Control System/Subsystem/position_control/vx  ==
  x : Inport
  reset_i : Inport  Port=2
  Derivative Gain : Gain  DisableCoverage=on  Gain=Kvxd
  Discrete Derivative : simulink/Discrete/Discrete Derivative  gainval=1.0  ICPrevScaledInput=0.0  OutMin=[]  OutMax=[]  OutDataType=fixdt(1, 16)  OutScaling=2^-10  DoSatur=off
  Discrete-Time Integrator : DiscreteIntegrator  ExternalReset=level  InitialConditionSetting=State (most efficient)  SampleTime=-1  LimitOutput=on  UpperSaturationLimit=Saturation_I_ah  LowerSaturationLimit=-Saturation_I_ah  ICPrevOutput=DiscIntNeverNeededParam  ICPrevScaledInput=DiscIntNeverNeededParam
  Gain : Gain  Gain=Kvxp
  Integral Gain : Gain  DisableCoverage=on  Gain=Kvxi
  Sum : Sum  Inputs=+++
  y : Outport  InitialOutput=0
  wires:
  x/1 -> Gain/1, Integral Gain/1, Derivative Gain/1
  Integral Gain/1 -> Discrete-Time Integrator/1
  Derivative Gain/1 -> Discrete Derivative/1
  Gain/1 -> Sum/1
  Sum/1 -> y/1
  Discrete Derivative/1 -> Sum/3
  Discrete-Time Integrator/1 -> Sum/2
  reset_i/1 -> Discrete-Time Integrator/2

== system ModeSwitch_FLY/Control System/Subsystem/position_control/vy  ==
  x : Inport
  reset_i : Inport  Port=2
  Derivative Gain : Gain  DisableCoverage=on  Gain=Kvyd
  Discrete Derivative : simulink/Discrete/Discrete Derivative  gainval=1.0  ICPrevScaledInput=0.0  OutMin=[]  OutMax=[]  OutDataType=fixdt(1, 16)  OutScaling=2^-10  DoSatur=off
  Discrete-Time Integrator : DiscreteIntegrator  ExternalReset=level  InitialConditionSetting=State (most efficient)  SampleTime=-1  LimitOutput=on  UpperSaturationLimit=Saturation_I_ah  LowerSaturationLimit=-Saturation_I_ah  ICPrevOutput=DiscIntNeverNeededParam  ICPrevScaledInput=DiscIntNeverNeededParam
  Gain : Gain  Gain=Kvyp
  Integral Gain : Gain  DisableCoverage=on  Gain=Kvyi
  Sum : Sum  Inputs=+++
  y : Outport  InitialOutput=0
  wires:
  x/1 -> Gain/1, Integral Gain/1, Derivative Gain/1
  Integral Gain/1 -> Discrete-Time Integrator/1
  Derivative Gain/1 -> Discrete Derivative/1
  Gain/1 -> Sum/1
  Sum/1 -> y/1
  Discrete Derivative/1 -> Sum/3
  Discrete-Time Integrator/1 -> Sum/2
  reset_i/1 -> Discrete-Time Integrator/2

== system ModeSwitch_FLY/Control System/Subsystem/position_control/vz  ==
  x : Inport
  reset_i : Inport  Port=2
  Derivative Gain : Gain  DisableCoverage=on  Gain=Kvzd
  Discrete Derivative : simulink/Discrete/Discrete Derivative  gainval=1.0  ICPrevScaledInput=0.0  OutMin=[]  OutMax=[]  OutDataType=fixdt(1, 16)  OutScaling=2^-10  DoSatur=off
  Discrete-Time Integrator : DiscreteIntegrator  ExternalReset=level  InitialConditionSetting=State (most efficient)  SampleTime=-1  LimitOutput=on  UpperSaturationLimit=Saturation_I_az  LowerSaturationLimit=-Saturation_I_az  ICPrevOutput=DiscIntNeverNeededParam  ICPrevScaledInput=DiscIntNeverNeededParam
  Gain : Gain  Gain=Kvzp
  Integral Gain : Gain  DisableCoverage=on  Gain=Kvzi
  Sum : Sum  Inputs=+++
  y : Outport  InitialOutput=0
  wires:
  Discrete-Time Integrator/1 -> Sum/2
  Discrete Derivative/1 -> Sum/3
  Sum/1 -> y/1
  Gain/1 -> Sum/1
  Derivative Gain/1 -> Discrete Derivative/1
  Integral Gain/1 -> Discrete-Time Integrator/1
  x/1 -> Derivative Gain/1, Integral Gain/1, Gain/1
  reset_i/1 -> Discrete-Time Integrator/2

== matlab function ModeSwitch_FLY/Control System/InputConditioning/deadzone2 ==
  data: u input; y output
function y = fcn(u)
%Function description:
%  Control the range of the remote control input from RCMin to RCMax, and
%  set a dead zone with a dead zone size of ±deadZone. The output y is
%  normalized to 0~1.You can get the RC calibration parameters in QGC.
RCMin = 1100;
RCMax = 1900;
RCMid = (RCMin + RCMax)/2;
deadZoneRate = 0.05;
deadZone = deadZoneRate*(RCMax - RCMin);
k = 1/(RCMax - RCMid - deadZone);
% saturation
if(u < RCMin)
    u = RCMin;
elseif(u > RCMax)
    u = RCMax;
end
% dead zone and normalize
 if(u > RCMid + deadZone)
    y = (u-RCMid - deadZone)*k;
 elseif(u < RCMid - deadZone)
     y = (u - RCMid + deadZone)*k;
 else
     y = 0;
 end

 end

== matlab function ModeSwitch_FLY/Control System/InputConditioning/deadzone3 ==
  data: u input; y output
function y = fcn(u)
%Function description:
%  Control the range of the remote control input from RCMin to RCMax, and
%  set a dead zone with a dead zone size of ±deadZone. The output y is
%  normalized to 0~1.You can get the RC calibration parameters in QGC.
RCMin = 1100;
RCMax = 1900;
RCMid = (RCMin + RCMax)/2;
deadZoneRate = 0.05;
deadZone = deadZoneRate*(RCMax - RCMin);
k = 1/(RCMax - RCMid - deadZone);
% saturation
if(u < RCMin)
    u = RCMin;
elseif(u > RCMax)
    u = RCMax;
end
% dead zone and normalize
 if(u > RCMid + deadZone)
    y = (u-RCMid - deadZone)*k;
 elseif(u < RCMid - deadZone)
     y = (u - RCMid + deadZone)*k;
 else
     y = 0;
 end

 end

== matlab function ModeSwitch_FLY/Control System/InputConditioning/deadzone1 ==
  data: u input; y output
function y = fcn(u)
%Function description:
%  Control the range of the remote control input from RCMin to RCMax, and
%  set a dead zone with a dead zone size of ±deadZone. The output y is
%  normalized to 0~1.You can get the RC calibration parameters in QGC.
RCMin = 1100;
RCMax = 1900;
RCMid = (RCMin + RCMax)/2;
deadZoneRate = 0.05;
deadZone = deadZoneRate*(RCMax - RCMin);
k = 1/(RCMax - RCMid - deadZone);
% saturation
if(u < RCMin)
    u = RCMin;
elseif(u > RCMax)
    u = RCMax;
end
% dead zone and normalize
 if(u > RCMid + deadZone)
    y = (u-RCMid - deadZone)*k;
 elseif(u < RCMid - deadZone)
     y = (u - RCMid + deadZone)*k;
 else
     y = 0;
 end

 end

== matlab function ModeSwitch_FLY/Control System/InputConditioning1/deadzone1 ==
  data: u input; y output
function y = fcn(u)
%Function description:
%  Control the range of the remote control input from RCMin to RCMax, and
%  set a dead zone with a dead zone size of ±deadZone. The output y is
%  normalized to 0~1.You can get the RC calibration parameters in QGC.
RCMin = 1100;
RCMax = 1900;
RCMid = (RCMin + RCMax)/2;
deadZoneRate = 0.05;
deadZone = deadZoneRate*(RCMax - RCMin);
k = 1/(RCMax - RCMid - deadZone);
% saturation
if(u < RCMin)
    u = RCMin;
elseif(u > RCMax)
    u = RCMax;
end
% dead zone and normalize
 if(u > RCMid + deadZone)
    y = (u-RCMid - deadZone)*k;
 elseif(u < RCMid - deadZone)
     y = (u - RCMid + deadZone)*k;
 else
     y = 0;
 end

 end

== matlab function ModeSwitch_FLY/Control System/InputConditioning1/deadzone2 ==
  data: u input; y output
function y = fcn(u)
%Function description:
%  Control the range of the remote control input from RCMin to RCMax, and
%  set a dead zone with a dead zone size of ±deadZone. The output y is
%  normalized to 0~1.You can get the RC calibration parameters in QGC.
RCMin = 1100;
RCMax = 1900;
RCMid = (RCMin + RCMax)/2;
deadZoneRate = 0.05;
deadZone = deadZoneRate*(RCMax - RCMin);
k = 1/(RCMax - RCMid - deadZone);
% saturation
if(u < RCMin)
    u = RCMin;
elseif(u > RCMax)
    u = RCMax;
end
% dead zone and normalize
 if(u > RCMid + deadZone)
    y = (u-RCMid - deadZone)*k;
 elseif(u < RCMid - deadZone)
     y = (u - RCMid + deadZone)*k;
 else
     y = 0;
 end

 end

== matlab function ModeSwitch_FLY/Control System/InputConditioning1/deadzone3 ==
  data: u input; y output
function y = fcn(u)
%Function description:
%  Control the range of the remote control input from RCMin to RCMax, and
%  set a dead zone with a dead zone size of ±deadZone. The output y is
%  normalized to 0~1.You can get the RC calibration parameters in QGC.
RCMin = 1100;
RCMax = 1900;
RCMid = (RCMin + RCMax)/2;
deadZoneRate = 0.05;
deadZone = deadZoneRate*(RCMax - RCMin);
k = 1/(RCMax - RCMid - deadZone);
% saturation
if(u < RCMin)
    u = RCMin;
elseif(u > RCMax)
    u = RCMax;
end
% dead zone and normalize
 if(u > RCMid + deadZone)
    y = (u-RCMid - deadZone)*k;
 elseif(u < RCMid - deadZone)
     y = (u - RCMid + deadZone)*k;
 else
     y = 0;
 end

 end

== matlab function ModeSwitch_FLY/Control System/MATLAB Function1 ==
  data: ch5 input; control_mode output
function control_mode  = fcn(ch5)
%Function description:
%  Map the remote control CH5 channel to control mode
%input:
%  ch5: Remote control CH5 channel input
%  control_mode: Custom control mode
%  0: stablelize mode；1: height control mode; 2: position control mode
if ch5 < 1400
    control_mode = int8(0);
elseif ch5 < 1600
    control_mode = int8(1);
else
    control_mode = int8(2);
end

== matlab function ModeSwitch_FLY/Control System/Subsystem/position_control/MATLAB Function ==
  data: eax input; eay input; psi input; phi output; theta output
function [phi, theta] = fcn(eax, eay, psi)
%Function description:
%  Convert the desired horizontal acceleration to the desired attitude angle
%Input:
%  eax, eaxy: desired horizontal acceleration
%  psi: yaw
%Output:
%  phi, theta: desired roll angle and desired pitch angle
g = 9.8;
phi = (-sin(psi)*eax + cos(psi)*eay)/g;
theta = (-cos(psi)*eax - sin(psi)*eay)/g;

== matlab function ModeSwitch_FLY/Control System/InputConditioning1/deadzone4 ==
  data: u input; y output
function y = fcn(u)
%Function description:
%  Control the range of the remote control input from RCMin to RCMax, and
%  set a dead zone with a dead zone size of ±deadZone. The output y is
%  normalized to 0~1.You can get the RC calibration parameters in QGC.
RCMin = 1100;
RCMax = 1900;
RCMid = (RCMin + RCMax)/2;
deadZoneRate = 0.05;
deadZone = deadZoneRate*(RCMax - RCMin);
k = 1/(RCMax - RCMid - deadZone);
% saturation
if(u < RCMin)
    u = RCMin;
elseif(u > RCMax)
    u = RCMax;
end
% dead zone and normalize
 if(u > RCMid + deadZone)
    y = (u-RCMid - deadZone)*k;
 elseif(u < RCMid - deadZone)
     y = (u - RCMid + deadZone)*k;
 else
     y = 0;
 end

 end

== matlab function ModeSwitch_FLY/Control System/MATLAB Function2 ==
  data: mode input; vxd input; vyd input; vx_d output; vy_d output; vz_d output; vzd input; x input; y input; z input; vx input; vy input; vz input; x_d output; y_d output; z_d output
function [vx_d, vy_d, vz_d, x_d, y_d, z_d] = fcn(mode, vxd, vyd, vzd, x, y, z, vx, vy, vz)
%Function description:
%  Mode switch implementation.
%Input:
%  mode
%  vxd, vyd, vzd: The desired velocity specified by the remote control
%  x, y, z: current position
%  vx, vy,vz: current velocity
%Output:
%  vx_d, vy_d, vz_d, x_d, y_d, z_d: desired velocity and position
persistent x1;
if isempty(x1)
    x1 = 0;
end
persistent y1;
if isempty(y1)
    y1 = 0;
end
persistent z1;
if isempty(z1)
    z1 = z;
end
persistent hold_x_flag;
if isempty(hold_x_flag)
    hold_x_flag = 0;
end
persistent hold_y_flag;
if isempty(hold_y_flag)
    hold_y_flag = 0;
end
persistent hold_z_flag;
if isempty(hold_z_flag)
    hold_z_flag = 0;
end
if mode == int8(0)
    x1 = x; y1 = y; z1 = z;
    vx_d = vx; vy_d = vy; vz_d = vz;
elseif mode == int8(1)
    x1 = x; y1 = y;
    vx_d = vx; vy_d = vy;
    
    if abs(vzd) < 0.001 && abs(vz) < 6
        hold_z = 1;
    else
         hold_z = 0;
        hold_z_flag = 0;
    end
    if (hold_z > 0.5) && (hold_z_flag < 0.5)
        z1 = z;
        hold_z_flag = 1;
    end
    if hold_z < 0.5
        z1 = z;
        hold_z_flag = 0;
    end
    vz_d = vzd;
else
    if abs(vxd) < 0.001 && abs(vx) < 8
        hold_x = 1;
    else
         hold_x = 0;
         hold_x_flag = 0;
    end
    if abs(vyd) < 0.001 && abs(vy) < 8
         hold_y = 1;
    else
         hold_y = 0;
        hold_y_flag = 0;
    end
    if abs(vzd) < 0.001 && abs(vz) < 6
        hold_z = 1;
    else
         hold_z = 0;
         hold_z_flag = 0;
    end

    if (hold_x > 0.5) && (hold_x_flag < 0.5)
            x1 = x;
            hold_x_flag = 1;
    end
    if (hold_y > 0.5) && (hold_y_flag < 0.5)
         y1 = y;
        hold_y_flag = 1;
    end
% throttle in the middle position, hold the height
    if (hold_z > 0.5) && (hold_z_flag < 0.5)
        z1 = z;
        hold_z_flag = 1;
    end
%When the RC sticks(CH1, CH2, CH3, CH4) deviate from the middle dead zone range, the position is the current position. 
%The position controller only works with the velocity loop
    if hold_x < 0.5
        x1 = x;
         hold_x_flag = 0;
    end
    if hold_y < 0.5
        y1 = y;
        hold_y_flag = 0;
    end
    if hold_z < 0.5
        z1 = z;
        hold_z_flag = 0;
    end
    vx_d = vxd; vy_d = vyd; vz_d = vzd;
end

x_d = x1;
y_d = y1;
z_d = z1;

== matlab function ModeSwitch_FLY/quat2eul ==
  data: q input; phi output; theta output; psi output
function [phi,theta,psi] = quat2eul(q)
% Conversion from Quaternion to Euler angles based on the PX4 Firmware
% v1.6.5 release.
% 
% Quaternion -> DCM -> Euler Angles
% INPUT:
%   q: Quaternion vector of the format: (a + bi + cj + dk)
% OUTPUT:
%   [phi,theta,psi]: Euler angles in radians.
% 
 
    a = q(1);
    b = q(2);
    c = q(3);
    d = q(4);

    aSq = a*a;
    bSq = b*b;
    cSq = c*c;
    dSq = d*d;

    d_pi2 = pi/2;

    % quaternion_to_dcm
    dcm00 = aSq + bSq - cSq - dSq;
    % dcm01 = 2*(b*c - a*d);
    dcm02 = 2*(a*c + b*d);
    dcm10 = 2*(b*c + a*d);
    % dcm11 = aSq - bSq + cSq - dSq;
    dcm12 = 2*(c*d - a*b);
    dcm20 = 2*(b*d - a*c);
    dcm21 = 2*(a*b + c*d);
    dcm22 = aSq - bSq - cSq + dSq;

    % dcm_to_euler
    theta = asin(-dcm20);
    if abs(theta - d_pi2) < 1.0e-3
        phi = single(0.0);
        psi = atan2(dcm12, dcm02);
    elseif abs(theta + d_pi2) < 1.0e-3
        phi = single(0.0);
        psi = atan2(-dcm12, -dcm02);
    else
        phi = atan2(dcm21, dcm22);
        psi = atan2(dcm10, dcm00);
    end

end

== matlab function ModeSwitch_FLY/Control System/Subsystem/pwm_out2 ==
  data: Roll input; M1 output; Pitch input; Yaw input; Thrust input; M2 output; M3 output; M4 output
function [M1, M2, M3, M4] = motor_mixer(Roll, Pitch, Yaw, Thrust)
%Function description:
%  Control allocation. The quadrotor type is X-configuration,
%  and the airframe is as follows:
%3↓   1↑
 %  \ /
 %  / \
 %2↑   4↓
%Input：
%  Roll, Pitch, Yaw: attitude controller output.
%  Thrust

idle_PWM = 1000;
scale = 1000;

M1 = (Thrust - Roll + Pitch + Yaw) * scale + idle_PWM;
M2 = (Thrust + Roll - Pitch + Yaw) * scale + idle_PWM;
M3 = (Thrust + Roll + Pitch - Yaw) * scale + idle_PWM;
M4 = (Thrust - Roll - Pitch - Yaw) * scale + idle_PWM;

== matlab function ModeSwitch_FLY/Control System/MATLAB Function3 ==
  data: mode input; reset_i output; ch3 input
function reset_i = fcn(mode, ch3)
%Function description:
%  reset Integral when throttle < 1250
if ch3 < 1250
    reset_i = [1 1 1 1];
elseif mode == 0
    reset_i = [0 0 1 1];
elseif mode == 1
    reset_i = [0 0 1 0];
else
    reset_i = [0 0 0 0];
end

== matlab function ModeSwitch_FLY/Control System/InputConditioning1/f1 ==
  data: in input; y output; hover input
function y = thr_curve(in, hover)
%Function description:
%  throttle curve. When the throttle is in the middle position, the output
%  is hovering throttle value.
%Input:
%  in: normalized throttle, range from 0 to 1
%  hover: hovering throttle value
%Output:
%  y: processed throttle value
if in < 0.5
	y=2 * in * hover;
else
	y=hover + 2 * (in - 0.5) * (1.0 - hover);
end
